simulink model "inverseDynamicsStandingTest"  (Simulink 7.7)
settings: Solver=FixedStepDiscrete  StartTime=0.0  StopTime=1000  FixedStep=0.01  RelTol=1e-3
PreLoadFcn:
  | robotName = 'icubGazeboSim';
  | localName = 'SimulinkiCubGazeboSim';
InitFcn:
  | robotName = 'icubGazeboSim';
  | localName = 'SimulinkiCubGazeboSim';
libraries: WBCLibrary x14, utility x1
settings Model: Creator=iron  LastModifiedBy=iron

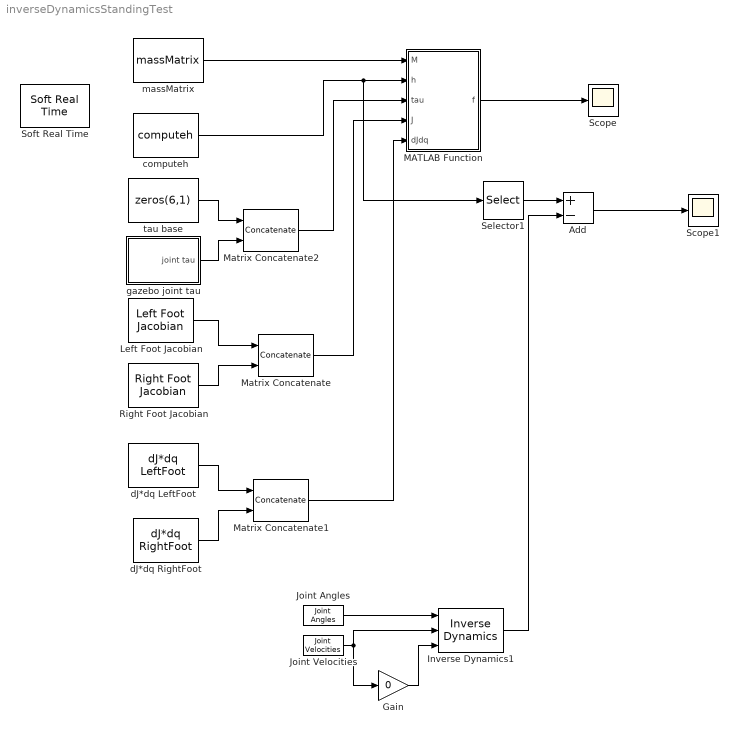
== system inverseDynamicsStandingTest ==
  Add : Sum  Inputs=+-
  Gain : Gain  Gain=0
  Inverse Dynamics1 : WBCLibrary/wholeBodyModel/Dynamics/Inverse Dynamics  SystemSampleTime=-1  robotName=robotName  localName=localName
  Joint Angles : WBCLibrary/wholeBodyStates/Joint Angles  SystemSampleTime=-1  robotName=robotName  localName=localName
  Joint Velocities : WBCLibrary/wholeBodyStates/Joint Velocities  SystemSampleTime=-1  robotName=robotName  localName=localName
  Left Foot Jacobian : WBCLibrary/wholeBodyModel/Jacobians/Left Foot Jacobian  SystemSampleTime=-1  robotName=robotName  localName=localName
  MATLAB Function : Stateflow chart  TreatAsAtomicUnit=on
  Matrix Concatenate : Concatenate  Mode=Multidimensional array
  Matrix Concatenate1 : Concatenate  Mode=Multidimensional array
  Matrix Concatenate2 : Concatenate  Mode=Multidimensional array
  Right Foot Jacobian : WBCLibrary/wholeBodyModel/Jacobians/Right Foot Jacobian  SystemSampleTime=-1  robotName=robotName  localName=localName
  Scope : Scope
      settings: YMin=-250  YMax=25
  Scope1 : Scope
      settings: YMin=-0.0025  YMax=0.025
  Selector1 : Selector  InputPortWidth=31  IndexOptions=Index vector (dialog)  Indices=[7:31]  OutputSizes=1
  Soft Real Time : utility/Soft Real Time  x=0.01
  computeh : WBCLibrary/wholeBodyModel/Dynamics/computeh  SystemSampleTime=-1  val=7  robotname=robotName  localname=localName
  dJ*dq LeftFoot : WBCLibrary/wholeBodyModel/Dynamics/dJ*dq LeftFoot  SystemSampleTime=-1  val=9  robotName=robotName  localName=localName
  dJ*dq RightFoot : WBCLibrary/wholeBodyModel/Dynamics/dJ*dq RightFoot  SystemSampleTime=-1  val=9  robotName=robotName  localName=localName
  gazebo joint tau : Subsystem
  massMatrix : WBCLibrary/wholeBodyModel/Dynamics/massMatrix  SystemSampleTime=-1  val=8  robotname=robotName  localname=localName
  tau base : Constant  Value=zeros(6,1)
  wires:
  massMatrix/1 -> MATLAB Function/1(M)
  computeh/1 -> MATLAB Function/2(h), Selector1/1
  Left Foot Jacobian/1 -> Matrix Concatenate/1
  Right Foot Jacobian/1 -> Matrix Concatenate/2
  Matrix Concatenate/1 -> MATLAB Function/4(J)
  dJ*dq LeftFoot/1 -> Matrix Concatenate1/1
  dJ*dq RightFoot/1 -> Matrix Concatenate1/2
  Matrix Concatenate1/1 -> MATLAB Function/5(dJdq)
  MATLAB Function/1(f) -> Scope/1
  tau base/1 -> Matrix Concatenate2/1
  gazebo joint tau/1(joint tau) -> Matrix Concatenate2/2
  Matrix Concatenate2/1 -> MATLAB Function/3(tau)
  Joint Velocities/1 -> Gain/1, Inverse Dynamics1/2
  Gain/1 -> Inverse Dynamics1/3
  Joint Angles/1 -> Inverse Dynamics1/1
  Add/1 -> Scope1/1
  Selector1/1 -> Add/1
  Inverse Dynamics1/1 -> Add/2

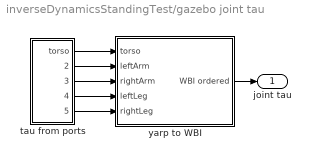
== system inverseDynamicsStandingTest/gazebo joint tau ==
  tau from ports : Subsystem
  yarp to WBI : Subsystem
  joint tau : Outport
  wires:
  tau from ports/2(leftArm) -> yarp to WBI/2(leftArm)
  tau from ports/1(torso) -> yarp to WBI/1(torso)
  tau from ports/5(rightLeg) -> yarp to WBI/5(rightLeg)
  tau from ports/3(rightArm) -> yarp to WBI/3(rightArm)
  tau from ports/4(leftLeg) -> yarp to WBI/4(leftLeg)
  yarp to WBI/1(WBI ordered) -> joint tau/1

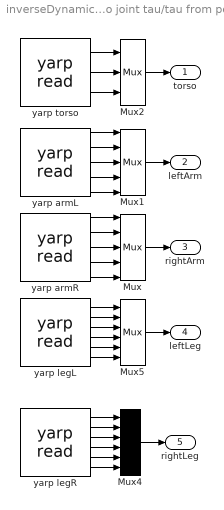
== system inverseDynamicsStandingTest/gazebo joint tau/tau from ports ==
  Mux : Mux  Inputs=5
  Mux1 : Mux  Inputs=5
  Mux2 : Mux  Inputs=3
  Mux4 : Mux  Inputs=6
  Mux5 : Mux  Inputs=6
  yarp armL : WBCLibrary/Utilities/yarp read  from='/icubGazeboSim/left_arm/analog:o/torques'  to='/tmp2:i'  num=5
  yarp armR : WBCLibrary/Utilities/yarp read  from='/icubGazeboSim/right_arm/analog:o/torques'  to='/tmp3:i'  num=5
  yarp legL : WBCLibrary/Utilities/yarp read  from='/icubGazeboSim/left_leg/analog:o/torques'  to='/tmp4:i'  num=6
  yarp legR : WBCLibrary/Utilities/yarp read  from='/icubGazeboSim/right_leg/analog:o/torques'  to='/tmp5:i'  num=6
  yarp torso : WBCLibrary/Utilities/yarp read  from='/icubGazeboSim/torso/analog:o/torques'  to='/tmp1:i'  num=3
  torso : Outport
  leftArm : Outport  Port=2
  rightArm : Outport  Port=3
  leftLeg : Outport  Port=4
  rightLeg : Outport  Port=5
  wires:
  yarp armR/1 -> Mux/1
  yarp armR/2 -> Mux/2
  yarp armR/3 -> Mux/3
  yarp armR/4 -> Mux/4
  yarp armR/5 -> Mux/5
  yarp armL/1 -> Mux1/1
  yarp armL/2 -> Mux1/2
  yarp armL/3 -> Mux1/3
  yarp armL/4 -> Mux1/4
  yarp armL/5 -> Mux1/5
  yarp torso/1 -> Mux2/1
  yarp torso/2 -> Mux2/2
  yarp torso/3 -> Mux2/3
  yarp legL/1 -> Mux5/1
  yarp legL/2 -> Mux5/2
  yarp legL/3 -> Mux5/3
  yarp legL/4 -> Mux5/4
  yarp legL/5 -> Mux5/5
  yarp legL/6 -> Mux5/6
  yarp legR/1 -> Mux4/1
  yarp legR/2 -> Mux4/2
  yarp legR/3 -> Mux4/3
  yarp legR/4 -> Mux4/4
  yarp legR/5 -> Mux4/5
  yarp legR/6 -> Mux4/6
  Mux2/1 -> torso/1
  Mux1/1 -> leftArm/1
  Mux/1 -> rightArm/1
  Mux5/1 -> leftLeg/1
  Mux4/1 -> rightLeg/1

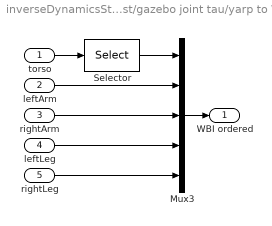
== system inverseDynamicsStandingTest/gazebo joint tau/yarp to WBI ==
  torso : Inport
  leftArm : Inport  Port=2
  rightArm : Inport  Port=3
  leftLeg : Inport  Port=4
  rightLeg : Inport  Port=5
  Mux3 : Mux  Inputs=5
  Selector : Selector  InputPortWidth=3  IndexOptions=Index vector (dialog)  Indices=[3 2 1]  OutputSizes=1
  WBI ordered : Outport
  wires:
  Selector/1 -> Mux3/1
  torso/1 -> Selector/1
  leftArm/1 -> Mux3/2
  rightArm/1 -> Mux3/3
  Mux3/1 -> WBI ordered/1
  leftLeg/1 -> Mux3/4
  rightLeg/1 -> Mux3/5

== matlab function MATLAB Function ==
  data: M input double; f output double; h input double; tau input double; J input double; dJdq input double
function f = fcn(M, h, tau, J, dJdq)

% Francesco Nori
% Genova 6 Marzo 2014
% CODYCO project
%
% This code computes the forces f acting on a kinematic chain
% subject to a set of constraints. The kinematic chain dynamics
% are described as follows:
%
% M d2q + h + J' * f = tau  
%
% The constraints are described in a differential form:
%
% J dq = 0
%
% whose derivative is:
%
% dJ dq  + J d2q = 0
%

Minv = inv(M);
f = (J*Minv*J')\(J*Minv*(tau - h)+ dJdq);
